simulink subsystem "Send_Actuator_Cmds_Fixed_Wing"  (R2025a)
settings: Solver=VariableStepAuto  StartTime=0.0  StopTime=10.0  RelTol=1e-3
libraries: px4Peripheralslib x3
settings Model: Creator=gurt1  LastModifiedBy=gurt1
settings RTWCC: GPUComputeCapability=3.5

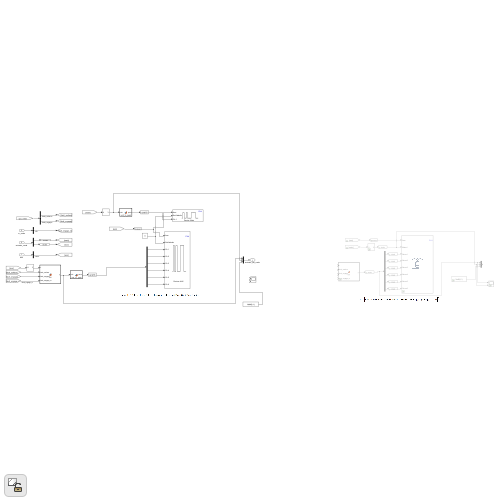
[thumbnail: Simulink's stored preview of the top-level diagram]
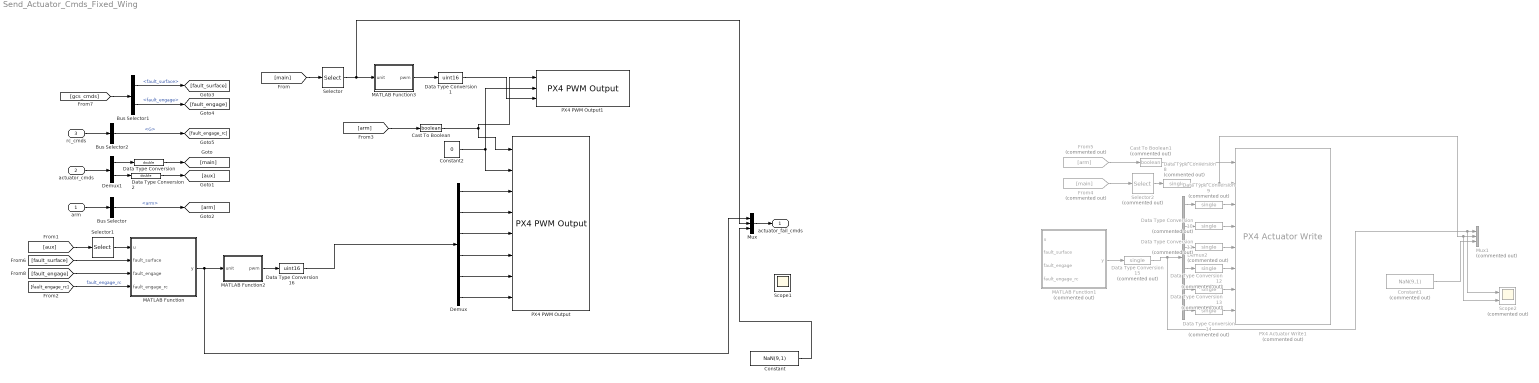
== system Send_Actuator_Cmds_Fixed_Wing ==
  arm : Inport
  actuator_cmds : Inport  Port=2
  rc_cmds : Inport  Port=3
  Bus Selector : BusSelector  OutputSignals=arm
  Bus Selector1 : BusSelector  OutputSignals=Fault.fault_surface,Fault.fault_engage
  Bus Selector2 : BusSelector  OutputSignals=switches.G
  Cast To Boolean : DataTypeConversion  OutDataTypeStr=boolean  SaturateOnIntegerOverflow=off  RndMeth=Floor
  Cast To Boolean1 : DataTypeConversion  Commented=on  OutDataTypeStr=boolean  SaturateOnIntegerOverflow=off  RndMeth=Floor
  Constant : Constant  Value=NaN(9,1)  OutDataTypeStr=double  SampleTime=-1
  Constant1 : Constant  Commented=on  Value=NaN(9,1)  OutDataTypeStr=single  SampleTime=-1
  Constant2 : Constant  Value=0  OutDataTypeStr=boolean  SampleTime=-1
  Data Type Conversion : DataTypeConversion  OutDataTypeStr=double  SaturateOnIntegerOverflow=off  RndMeth=Floor
  Data Type Conversion1 : DataTypeConversion  OutDataTypeStr=uint16  SaturateOnIntegerOverflow=off  RndMeth=Floor
  Data Type Conversion{8..15} (8 alike) : DataTypeConversion  Commented=on  OutDataTypeStr=single  SaturateOnIntegerOverflow=off  RndMeth=Floor
  Data Type Conversion16 : DataTypeConversion  OutDataTypeStr=uint16  SaturateOnIntegerOverflow=off  RndMeth=Floor
  Data Type Conversion2 : DataTypeConversion  OutDataTypeStr=double  SaturateOnIntegerOverflow=off  RndMeth=Floor
  Demux : Demux  Outputs=6
  Demux1 : Demux  Outputs=[8 8]
  Demux2 : Demux  Commented=on  Outputs=6
  From4 : From  Commented=on  GotoTag=main
  From5 : From  Commented=on  GotoTag=arm
  MATLAB Function : MATLAB Function  TreatAsAtomicUnit=on
  MATLAB Function1 : MATLAB Function  Commented=on  TreatAsAtomicUnit=on
  MATLAB Function2 : MATLAB Function  TreatAsAtomicUnit=on
  MATLAB Function3 : MATLAB Function  TreatAsAtomicUnit=on
  Mux : Mux  Inputs=3
  Mux1 : Mux  Commented=on  Inputs=3
  PX4 Actuator Write1 : px4Peripheralslib/PX4 Actuator Write  Commented=on  Motor1Enable=on  Motor2Enable=off  Motor3Enable=off  Motor4Enable=off  Motor5Enable=off  Motor6Enable=off  Motor7Enable=off  Motor8Enable=off  Motor9Enable=off  Motor10Enable=off  Motor11Enable=off  Motor12Enable=off  IsMotorArray=off  Servo1Enable=on  Servo2Enable=on  Servo3Enable=on  Servo4Enable=on  Servo5Enable=on  Servo6Enable=on  Servo7Enable=off  Servo8Enable=off  IsServoArray=off
  PX4 PWM Output : px4Peripheralslib/PX4 PWM Output  pwmDevice=AUX  pwmChannel1_=on  pwmChannel2_=on  pwmChannel3_=on  pwmChannel4_=on  pwmChannel5_=on  pwmChannel6_=on  pwmChannel7_=off  pwmChannel8_=off
  PX4 PWM Output1 : px4Peripheralslib/PX4 PWM Output  pwmDevice=Main  pwmChannel1_=on  pwmChannel2_=off  pwmChannel3_=off  pwmChannel4_=off  pwmChannel5_=off  pwmChannel6_=off  pwmChannel7_=off  pwmChannel8_=off
  Scope1 : Scope  NumInputPorts=2
      settings: ActiveDisplayYMinimum=-1  ActiveDisplayYMaximum=1  DataLoggingVariableName=ScopeData10
  Scope2 : Scope  Commented=on  NumInputPorts=2
      settings: ActiveDisplayYMinimum=-1  ActiveDisplayYMaximum=1  DataLoggingVariableName=ScopeData2
  Selector : Selector  InputPortWidth=8  IndexOptions=Index vector (dialog)  Indices=1  OutputSizes=1
  Selector1 : Selector  InputPortWidth=8  IndexOptions=Index vector (dialog)  Indices=[1:6]  OutputSizes=1
  Selector2 : Selector  Commented=on  InputPortWidth=8  IndexOptions=Index vector (dialog)  Indices=1  OutputSizes=1
  actuator_fail_cmds : Outport
  wires:
  Demux1/1 -> Data Type Conversion/1
  actuator_cmds/1 -> Demux1/1
  Demux1/2 -> Data Type Conversion2/1
  [arm] -> Cast To Boolean/1
  [main] -> Selector/1
  Selector/1 -> MATLAB Function3/1(unit), Mux/2
  [aux] -> Selector1/1
  Selector1/1 -> MATLAB Function/1(u)
  MATLAB Function3/1(pwm) -> Data Type Conversion1/1
  arm/1 -> Bus Selector/1
  Bus Selector/1 -> [arm]  "<arm>"
  [gcs_cmds] -> Bus Selector1/1
  Bus Selector1/1 -> [fault_surface]  "<fault_surface>"
  Bus Selector1/2 -> [fault_engage]  "<fault_engage>"
  [fault_surface] -> MATLAB Function/2(fault_surface)
  [fault_engage] -> MATLAB Function/3(fault_engage)
  Mux/1 -> actuator_fail_cmds/1
  Constant/1 -> Mux/3
  rc_cmds/1 -> Bus Selector2/1
  Bus Selector2/1 -> [fault_engage_rc]  "<G>"
  [fault_engage_rc] -> MATLAB Function/4(fault_engage_rc)  "fault_engage_rc"
  Data Type Conversion15/1 -> Scope2/1, Mux1/1, Demux2/1
  Constant1/1 -> Mux1/3
  MATLAB Function1/1(y) -> Data Type Conversion15/1
  Data Type Conversion12/1 -> PX4 Actuator Write1/6
  Demux2/4 -> Data Type Conversion12/1
  Data Type Conversion14/1 -> PX4 Actuator Write1/8
  Demux2/6 -> Data Type Conversion14/1
  Demux2/5 -> Data Type Conversion13/1
  Data Type Conversion13/1 -> PX4 Actuator Write1/7
  Cast To Boolean1/1 -> PX4 Actuator Write1/1
  Data Type Conversion8/1 -> Scope2/2, Mux1/2, PX4 Actuator Write1/2
  Data Type Conversion11/1 -> PX4 Actuator Write1/5
  Data Type Conversion10/1 -> PX4 Actuator Write1/4
  Data Type Conversion9/1 -> PX4 Actuator Write1/3
  Demux2/3 -> Data Type Conversion11/1
  Demux2/2 -> Data Type Conversion10/1
  Demux2/1 -> Data Type Conversion9/1
  Selector2/1 -> Data Type Conversion8/1
  From4/1 -> Selector2/1
  From5/1 -> Cast To Boolean1/1
  Cast To Boolean/1 -> PX4 PWM Output/1, PX4 PWM Output1/1
  Constant2/1 -> PX4 PWM Output/2, PX4 PWM Output1/2
  Data Type Conversion16/1 -> Demux/1
  MATLAB Function2/1(pwm) -> Data Type Conversion16/1
  MATLAB Function/1(y) -> MATLAB Function2/1(unit), Mux/1
  Data Type Conversion/1 -> [main]
  Data Type Conversion2/1 -> [aux]
  Data Type Conversion1/1 -> PX4 PWM Output1/3
  Demux/6 -> PX4 PWM Output/8
  Demux/5 -> PX4 PWM Output/7
  Demux/4 -> PX4 PWM Output/6
  Demux/3 -> PX4 PWM Output/5
  Demux/2 -> PX4 PWM Output/4
  Demux/1 -> PX4 PWM Output/3

== matlab function Send_Actuator_Cmds_Fixed_Wing/MATLAB Function1 ==
  data: u input; fault_surface input; y output; fault_engage input; fault_engage_rc input
function y = fcn(u, fault_surface, fault_engage, fault_engage_rc)

if fault_engage_rc == 0% || fault_engage == 1
    u(fault_surface) = 0;
    y = u;
else
    y = u;
end

== matlab function Send_Actuator_Cmds_Fixed_Wing/MATLAB Function3 ==
  data: unit input; pwm output
%% unit_to_pwm
% DESCRIPTION: 
%   This function reads in a vector and maps the input from 0 to 1 to the range 
%   of 1000 to 2000. It also checks if any input values are -1 or NaN, and if so, 
%   sets the corresponding output value to 800.
%
% INPUTS: 
%   u   - (Nx1) Input vector with values to be mapped
%
% OUTPUTS:
%   y   - (Nx1) Output vector with mapped PWM values (1000 to 2000 or 800 for invalid inputs)
% 
% WRITTEN BY:
%   Garrett D. Asper
%   Virginia Tech
%   Email: garrettasper@vt.edu
%
% HISTORY:
%   16 SEP 2024 - Created and debugged, GDA
%
% NOMENCLATURE:                                  UNITS:
%   Not Applicable                                  Not Applicable

function pwm = unit_to_pwm(unit)

    % Map the input from 0 to 1 to 1000 to 2000
    pwm = unit*1000 + 1000;

    % Iterate through each value to apply constraints
    for i = 1:length(pwm)
        if isnan(unit(i)) || unit(i) == -1
            % Set the output to 800 for invalid inputs (-1 or NaN)
            pwm(i) = 800;
        elseif pwm(i) > 2000
            pwm(i) = 2000;
        elseif pwm(i) < 1000
            pwm(i) = 1000;
        end
    end

end

== matlab function Send_Actuator_Cmds_Fixed_Wing/MATLAB Function ==
  data: u input; fault_surface input; y output; fault_engage input; fault_engage_rc input
function y = fcn(u, fault_surface, fault_engage, fault_engage_rc)

if fault_engage_rc == 0% || fault_engage == 1
    u(fault_surface) = 0;
    y = u;
else
    y = u;
end

== matlab function Send_Actuator_Cmds_Fixed_Wing/MATLAB Function2 ==
  data: unit input; pwm output
%% unit_to_pwm
% DESCRIPTION: 
%   This function reads in a vector and maps the input from 0 to 1 to the range 
%   of 1000 to 2000. It also checks if any input values are -1 or NaN, and if so, 
%   sets the corresponding output value to 800.
%
% INPUTS: 
%   u   - (Nx1) Input vector with values to be mapped
%
% OUTPUTS:
%   y   - (Nx1) Output vector with mapped PWM values (1000 to 2000 or 800 for invalid inputs)
% 
% WRITTEN BY:
%   Garrett D. Asper
%   Virginia Tech
%   Email: garrettasper@vt.edu
%
% HISTORY:
%   16 SEP 2024 - Created and debugged, GDA
%
% NOMENCLATURE:                                  UNITS:
%   Not Applicable                                  Not Applicable

function pwm = unit_to_pwm(unit)

    % Map the input from 0 to 1 to 1000 to 2000
    unit = (unit+1)./2;
    pwm = unit*1000 + 1000;

    % Iterate through each value to apply constraints
    for i = 1:length(pwm)
        if isnan(unit(i)) || unit(i) == -1
            % Set the output to 800 for invalid inputs (-1 or NaN)
            pwm(i) = 800;
        elseif pwm(i) > 2000
            pwm(i) = 2000;
        elseif pwm(i) < 1000
            pwm(i) = 1000;
        end
    end

end
